simulink model "DC_speed_i_close_loop"  (R2020b)
settings: Solver=VariableStepAuto  StartTime=0.0  StopTime=5  RelTol=1e-3
undefined symbols (not defined in the file): D1, lagging, pulse
libraries: powerlib x8, simulink x7, powerlib_meascontrol x3
settings Model: Creator=JinYU  LastModifiedBy=JinYU
settings SolverCC: ZeroCrossAlgorithm=Adaptive
settings DebuggingCC: IgnoredZcDiagnostic=none

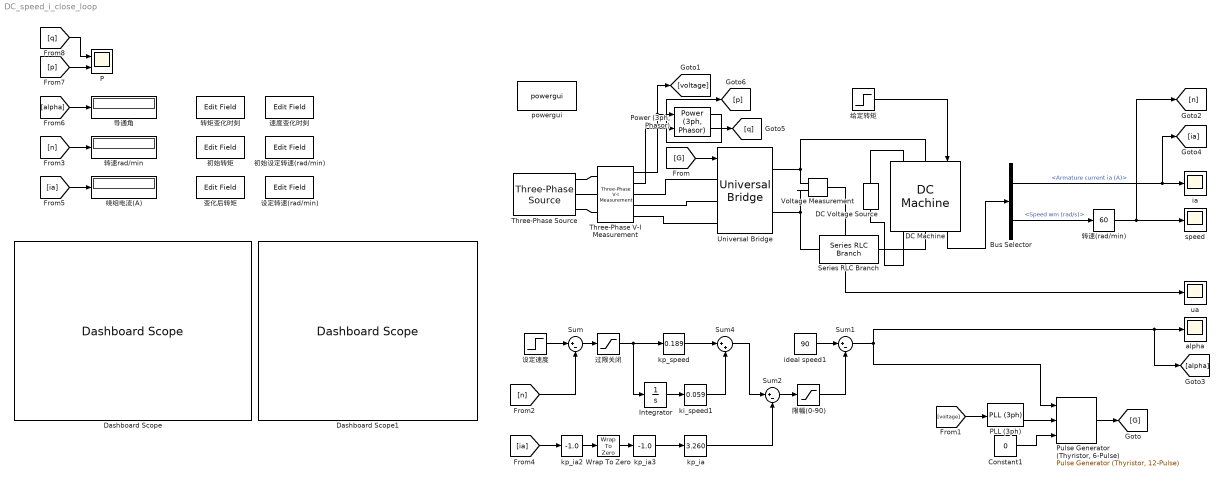
== system DC_speed_i_close_loop ==
  Bus Selector : BusSelector  OutputSignals=Armature current ia (A),Speed wm (rad/s)
  Constant1 : Constant  Value=0
  DC Machine : powerlib/Machines/DC Machine  PresetModel=No  MechanicalLoad=Torque TL  FieldType=Wound  ShowDetailedParameters=on  MeasurementBus=off  RLa="[ 0.6  0.012]"  RLf="[ 240  120]"  Laf=1.8  MachineConstant=Torque constant (N.m/A)  Ke=1.8  Kt=1.8  J=1  Bm=0  Tf=0  w0=40  Ifinit=0.625  TsPowergui=0  TsBlock=-1
  DC Voltage Source : powerlib/Electrical Sources/DC Voltage Source  Amplitude=150  Measurements=None
  Dashboard Scope : DashboardScope  Ymin=2000  Ymax=4000  ScaleAtStop=off
  Dashboard Scope1 : DashboardScope  Ymin=0  Ymax=20  ScaleAtStop=off
  Integrator : Integrator
  P : Scope  NumInputPorts=2
  PLL (3ph) : powerlib_meascontrol/PLL/PLL (3ph)  Fmin=45  Par_Init=[0, 50]  ParK=[180, 3200, 1]  TcD=1e-4  MaxRateChangeFreq=12  FilterCutOffFreq=25  Ts=0  AGC=on
  "Power (3ph, Phasor)" : powerlib_meascontrol/Measurements/Power (3ph, Phasor)
      settings: SourceProductBaseCode=PS
  "Pulse Generator (Thyristor, 6-Pulse)" : powerlib_meascontrol/Pulse & Signal Generators/Pulse Generator (Thyristor, 12-Pulse)  GenType=6-pulse  Delta=D1 (lagging)  pwidth=80  Double_Pulse=off  Ts=0
      settings: SourceProductBaseCode=PS
  Series RLC Branch : powerlib/Elements/Series RLC Branch  LConnTagsString=__new0  RConnTagsString=__new0  BranchType=L  Resistance=1  Inductance=1  SetiL0=off  InitialCurrent=0  Capacitance=1e-6  Setx0=off  InitialVoltage=0  Measurements=None
  Sum : Sum  Inputs=|+-
  Sum1 : Sum  Inputs=|+-
  Sum2 : Sum  Inputs=|+-
  Sum4 : Sum  Inputs=|++
  Three-Phase V-I Measurement : powerlib/Measurements/Three-Phase V-I Measurement  VoltageMeasurement=phase-to-ground  SetLabelV=off  LabelV=Vabc  Vpu=off  VpuLL=off  CurrentMeasurement=yes  SetLabelI=off  LabelI=Iabc  Ipu=off  Pbase=100e6  Vbase=500e3  OutputType=Complex  PhasorSimulation=off  PSBequivalent=0
  Three-Phase Source : powerlib/Electrical Sources/Three-Phase Source  InternalConnection=Yg  VoltagePhases=off  Voltage=400  PhaseAngle=0  Voltage_phases=[25e3 25e3 25e3]/sqrt(3)  PhaseAngles_phases=[0 -120 +120]  Frequency=50  NonIdealSource=on  SpecifyImpedance=off  Resistance=0.08929  Inductance=16.58e-3  ShortCircuitLevel=100e6  BaseVoltage=25e3  XRratio=7  BusType=swing  Pref=10e3  Qref=0  Prefabc=[10e3, 10e3, 10e3]  Qrefabc=[0, 0, 0]  Qmin=-inf  Qmax=inf
  Universal Bridge : powerlib/Power Electronics/Universal Bridge  Arms=3  SnubberResistance=1e5  SnubberCapacitance=inf  Device=Thyristors  Ron=1e-3  Lon=0  ForwardVoltages="[  0  0  ]"  ForwardVoltage=0  GTOparameters=[ 10e-6 , 20e-6 ]  IGBTparameters=[ 1e-6 , 2e-6 ]  Measurements=None  Measurements_2=None  converterType=Rectifier
  Voltage Measurement : powerlib/Measurements/Voltage Measurement  PhasorSimulation=off  OutputType=Complex  PSBequivalent=0
  Wrap To Zero : simulink/Discontinuities/Wrap To Zero  Threshold=-8
      settings: SourceProductBaseCode=SL
  alpha : Scope
  ia : Scope
  ideal speed1 : Constant  Value=90
  ki_speed1 : simulink/Math Operations/Slider Gain  gain=0.059  low=0.01  high=0.5
  kp_ia : simulink/Math Operations/Slider Gain  gain=3.260  low=2  high=5
  kp_ia2 : simulink/Math Operations/Slider Gain  gain=-1.0  low=-1  high=5
  kp_ia3 : simulink/Math Operations/Slider Gain  gain=-1.0  low=-1  high=5
  kp_speed : simulink/Math Operations/Slider Gain  gain=0.189  low=0  high=0.3
  powergui : powerlib/powergui  Priority=1  SimulationMode=Continuous  SampleTime=50e-6  frequency=60  Iterations=50  frequencyindice=50  Pbase=100e6  ErrMax=1e-4  UnitsV=kV  UnitsW=MW  buscounter=0  FunctionMessages=off  echomessages=off  EnableUseOfTLC=off  CurrentSourceSwitches=off  DisableSnubberDevices=off  DisableRonSwitches=off  DisableVfSwitches=off  DisplayEquations=off  AutomaticDiscreteSolvers=off  SolverType=Tustin/Backward Euler (TBE)  Interpol=off  ExternalGateDelay=off  methode=off  Ts=100  x0status=blocks  SPID=on  SwTol=0  HookPort=off  NonlinearTolerance=1e-4  nMaxIteration=100  ContinueOnMaxIteration=off  RestoreLinks=warning  ResistiveCurrentMeasurement=off  Frange=[0:2:500]  Ylog=off  Xlog=on  ShowGrid=off  save=off  variable=ZData  structure=0  ZoomFFT=off  StartTime=0.0  cycles=1  DisplayStyle=1  fundamental=60  FreqAxis=off  MaxFrequency=1000  frequencyindicesteady=1  RmsSteady=1  display=off
  speed : Scope
  ua : Scope
  初始设定转速(rad/min) : EditField  LabelPosition=Hide  ShowInitialText=on  Alignment=Center
  初始转矩 : EditField  LabelPosition=Hide  ShowInitialText=on  Alignment=Center
  变化后转矩 : EditField  LabelPosition=Hide  ShowInitialText=on  Alignment=Center
  导通角 : Display
  绕组电流(A) : Display
  给定转矩 : Step  Time=2.5  Before=1  SampleTime=0
  设定转速(rad/min) : EditField  LabelPosition=Hide  ShowInitialText=on  Alignment=Center
  设定速度 : Step  Time=5  Before=3000  After=2400  SampleTime=0
  转矩变化时刻 : EditField  LabelPosition=Hide  ShowInitialText=on  Alignment=Center
  转速(rad/min) : simulink/Math Operations/Slider Gain  gain=60  low=0  high=100
  转速rad/min : Display
  过限关闭 : Saturate  UpperLimit=300  LowerLimit=-300
  速度变化时刻 : EditField  LabelPosition=Hide  ShowInitialText=on  Alignment=Center
  限幅(0-90) : Saturate  UpperLimit=90  LowerLimit=0
  wires:
  DC Machine/1 -> Bus Selector/1
  Voltage Measurement/1 -> ua/1
  "Pulse Generator (Thyristor, 6-Pulse)"/1 -> [G]
  Three-Phase V-I Measurement/1 -> [voltage], "Power (3ph, Phasor)"/1
  PLL (3ph)/2 -> "Pulse Generator (Thyristor, 6-Pulse)"/2
  [voltage] -> PLL (3ph)/1
  Constant1/1 -> "Pulse Generator (Thyristor, 6-Pulse)"/3
  Sum1/1 -> "Pulse Generator (Thyristor, 6-Pulse)"/1, [alpha], alpha/1
  Bus Selector/1 -> [ia], ia/1  "<Armature current ia (A)>"
  ideal speed1/1 -> Sum1/1
  [n] -> Sum/2
  限幅(0-90)/1 -> Sum1/2
  [G] -> Universal Bridge/1
  Sum2/1 -> 限幅(0-90)/1
  Integrator/1 -> ki_speed1/1
  [n] -> 转速rad/min/1
  [ia] -> 绕组电流(A)/1
  kp_speed/1 -> Sum4/1
  ki_speed1/1 -> Sum4/2
  Sum4/1 -> Sum2/1
  设定速度/1 -> Sum/1
  转速(rad/min)/1 -> [n], speed/1
  Bus Selector/2 -> 转速(rad/min)/1  "<Speed wm (rad/s)>"
  给定转矩/1 -> DC Machine/1
  Sum/1 -> 过限关闭/1
  过限关闭/1 -> Integrator/1, kp_speed/1
  kp_ia/1 -> Sum2/2
  [ia] -> kp_ia2/1
  kp_ia2/1 -> Wrap To Zero/1
  Wrap To Zero/1 -> kp_ia3/1
  kp_ia3/1 -> kp_ia/1
  [alpha] -> 导通角/1
  [p] -> P/2
  [q] -> P/1
  Three-Phase V-I Measurement/2 -> "Power (3ph, Phasor)"/2
  "Power (3ph, Phasor)"/2 -> [q]
  "Power (3ph, Phasor)"/1 -> [p]
  connections:
  DC Voltage Source/RConn1 -- DC Machine/LConn2
  DC Machine/RConn2 -- DC Voltage Source/LConn1
  Universal Bridge/RConn1 -- DC Machine/LConn1 -- Voltage Measurement/LConn1
  Three-Phase Source/RConn1 -- Three-Phase V-I Measurement/LConn1
  Three-Phase Source/RConn2 -- Three-Phase V-I Measurement/LConn2
  Three-Phase Source/RConn3 -- Three-Phase V-I Measurement/LConn3
  Three-Phase V-I Measurement/RConn1 -- Universal Bridge/LConn1
  Three-Phase V-I Measurement/RConn2 -- Universal Bridge/LConn2
  Universal Bridge/LConn3 -- Three-Phase V-I Measurement/RConn3
  Series RLC Branch/LConn1 -- Voltage Measurement/LConn2 -- Universal Bridge/RConn2
  Series RLC Branch/RConn1 -- DC Machine/RConn1
